simulink model "SeguidorDeLineaPP"  (R2023b)
settings: Solver=FixedStepDiscrete  StartTime=0.0  StopTime=inf  FixedStep=0.01  RelTol=1e-3  EnableMultiTasking=on
model workspace (MAT data in the model file):
  baldosa = 0.48
  baldosa2 = 0.41
  d = 0.2625
settings Model: ExtModeTrigDuration=2  Creator=Usuario_UMA  LastModifiedBy=pablo
settings SolverCC: AlgebraicLoopSolver=TrustRegion  AutoInsertRateTranBlk=on
settings OptimizationCC: EnhancedBackFolding=on  PassReuseOutputArgsAs=Individual arguments  ZeroExternalMemoryAtStartup=off  ZeroInternalMemoryAtStartup=off  MaxStackSize=64  OptimizeBlockOrder=speed  DifferentSizesBufferReuse=on  EfficientTunableParamExpr=on
settings DebuggingCC: ParameterTunabilityLossMsg=error  UnconnectedInputMsg=warning  UnconnectedOutputMsg=warning  UnconnectedLineMsg=warning
settings HardwareCC: ProdBitPerInt=16  ProdBitPerPointer=16  ProdBitPerSizeT=16  ProdBitPerPtrDiffT=16  ProdLargestAtomicFloat=None  ProdWordSize=8  ProdHWDeviceType=Atmel->AVR  UseEmbeddedCoderFeatures=off  UseSimulinkCoderFeatures=off
settings ModelReferenceCC: EnableRefExpFcnMdlSchedulingChecks=on
settings SFSimCC: MATLABDynamicMemAlloc=off
settings RTWCC: Description=Embedded Coder  SystemTargetFile=ert.tlc  HardwareBoard=Arduino Mega 2560  TemplateMakefile=ert_default_tmf  Toolchain=Arduino AVR  BuildConfiguration=Faster Runs  DLArmComputeVersion=19.05
settings CodeAppCC: ForceParamTrailComments=on  IgnoreCustomStorageClasses=off  OperatorAnnotations=on  SimulinkDataObjDesc=on  SFDataObjDesc=on  MangleLength=10  InsertBlockDesc=on
settings ERTTargetCC: SupportContinuousTime=on  SupportNonInlinedSFcns=on  SupportVariableSizeSignals=on  ExtModeTransport=3  ExtModeStaticAlloc=on  ExtModeAutomaticAllocSize=off  ExtModeStaticAllocSize=2048  ExtModeMexFile=ext_xcp  ExtModeIntrfLevel=Level2 - Open

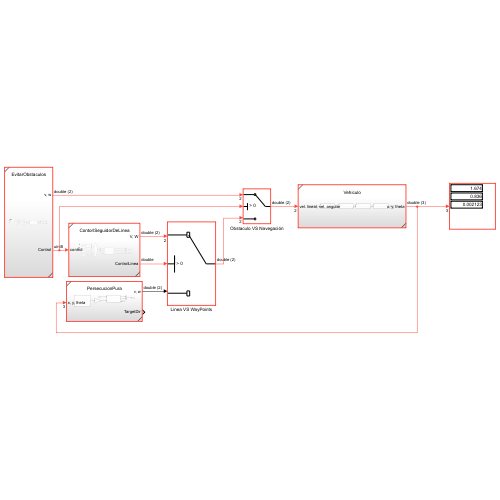
[thumbnail: Simulink's stored preview of the top-level diagram]
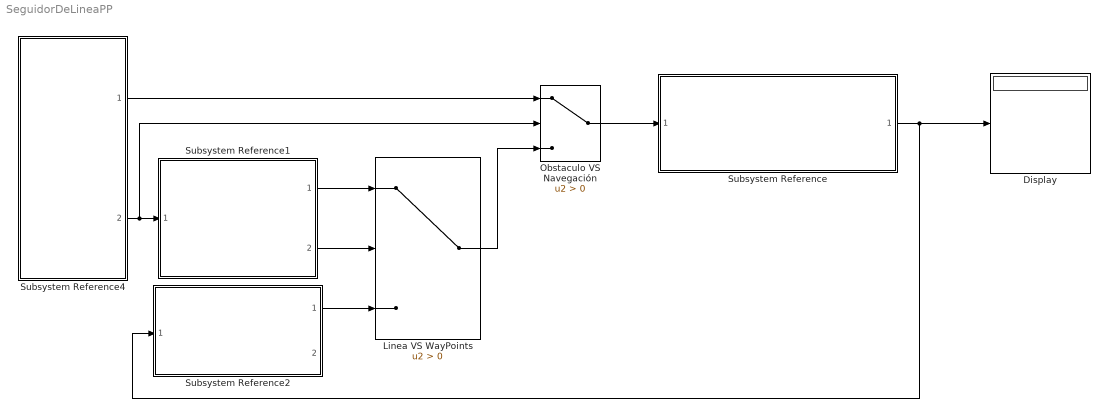
== system SeguidorDeLineaPP ==
  Display : Display
  Linea VS WayPoints : Switch  Criteria=u2 > Threshold  SaturateOnIntegerOverflow=off  InputSameDT=off
  Obstaculo VS Navegación : Switch  Criteria=u2 > Threshold  SaturateOnIntegerOverflow=off  InputSameDT=off
  Subsystem Reference : Subsystem  ReferencedSubsystem=Vehiculo
  Subsystem Reference1 : Subsystem  ReferencedSubsystem=ContorlSeguidorDeLinea
  Subsystem Reference2 : Subsystem  ReferencedSubsystem=PersecucionPura
  Subsystem Reference4 : Subsystem  ReferencedSubsystem=EvitarObstaculos
  wires:
  Obstaculo VS Navegación/1 -> Subsystem Reference/1
  Subsystem Reference1/1 -> Linea VS WayPoints/1
  Subsystem Reference/1 -> Subsystem Reference2/1, Display/1
  Linea VS WayPoints/1 -> Obstaculo VS Navegación/3
  Subsystem Reference4/2 -> Obstaculo VS Navegación/2, Subsystem Reference1/1
  Subsystem Reference4/1 -> Obstaculo VS Navegación/1
  Subsystem Reference1/2 -> Linea VS WayPoints/2
  Subsystem Reference2/1 -> Linea VS WayPoints/3
